simulink model "ITMBS_epushbtton_M0"  (R2023a)
settings: Solver=FixedStepDiscrete  StartTime=0.0  StopTime=10.0  FixedStep=0.05  RelTol=1e-3
libraries: legoev3lib x4
settings Model: Creator=kevin  LastModifiedBy=Sachin K S

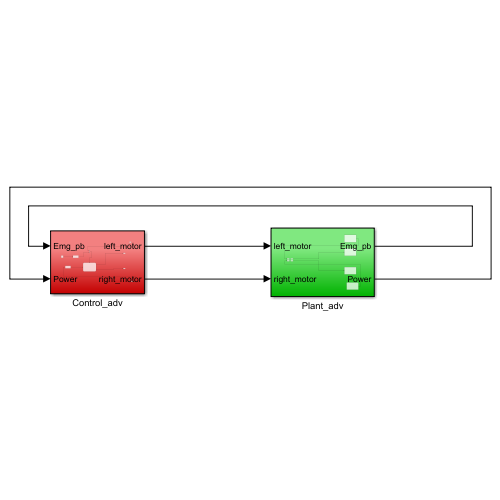
[thumbnail: Simulink's stored preview of the top-level diagram]
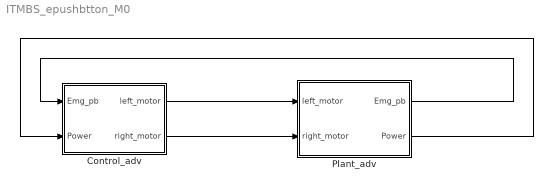
== system ITMBS_epushbtton_M0 ==
  Control_adv : Subsystem
  Plant_adv : Subsystem
  wires:
  Control_adv/1(left_motor) -> Plant_adv/1(left_motor)
  Control_adv/2(right_motor) -> Plant_adv/2(right_motor)
  Plant_adv/1(Emg_pb) -> Control_adv/1(Emg_pb)
  Plant_adv/2(Power) -> Control_adv/2(Power)

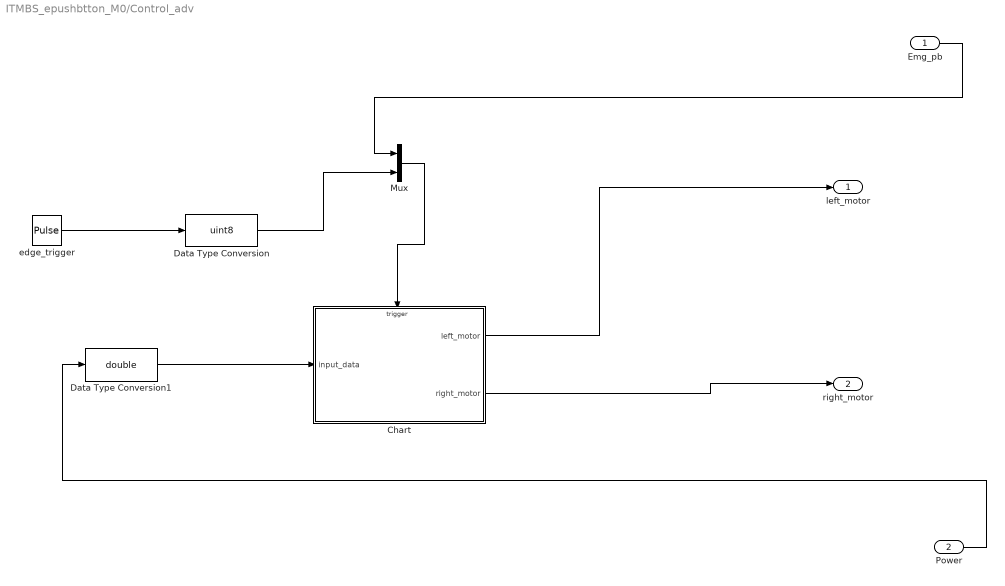
== system ITMBS_epushbtton_M0/Control_adv ==
  Emg_pb : Inport
  Power : Inport  Port=2
  Chart : Stateflow chart  TreatAsAtomicUnit=on
  Data Type Conversion : DataTypeConversion  OutDataTypeStr=uint8  SaturateOnIntegerOverflow=off  RndMeth=Floor
  Data Type Conversion1 : DataTypeConversion  OutDataTypeStr=double  SaturateOnIntegerOverflow=off  RndMeth=Floor
  Mux : Mux  Inputs=2
  edge_trigger : DiscretePulseGenerator  Period=3  PulseWidth=2  SampleTime=0.05
  left_motor : Outport
  right_motor : Outport  Port=2
  wires:
  Mux/1 -> Chart/Trigger
  edge_trigger/1 -> Data Type Conversion/1
  Chart/1(left_motor) -> left_motor/1
  Chart/2(right_motor) -> right_motor/1
  Data Type Conversion/1 -> Mux/2
  Data Type Conversion1/1 -> Chart/1(input_data)
  Power/1 -> Data Type Conversion1/1
  Emg_pb/1 -> Mux/1

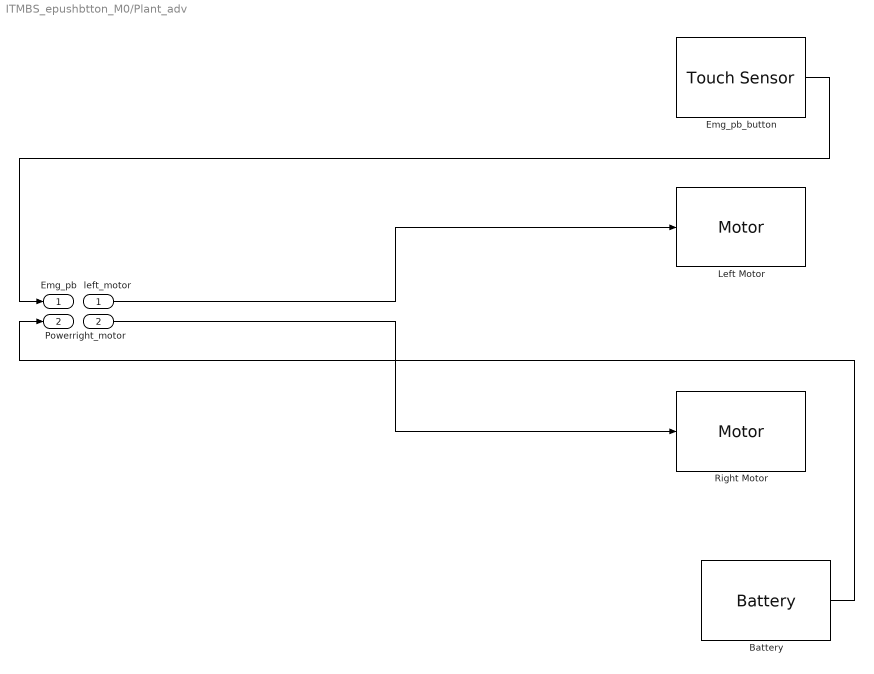
== system ITMBS_epushbtton_M0/Plant_adv ==
  left_motor : Inport
  right_motor : Inport  Port=2
  Battery : legoev3lib/Battery  SampleTime=0.1
  Emg_pb_button : legoev3lib/Touch Sensor  portNumber=1  sampleTime=0.1
  Left Motor : legoev3lib/Motor  sportNumber=A  sstopAction=Brake
  Right Motor : legoev3lib/Motor  sportNumber=A  sstopAction=Brake
  Emg_pb : Outport
  Power : Outport  Port=2
  wires:
  Emg_pb_button/1 -> Emg_pb/1
  left_motor/1 -> Left Motor/1
  right_motor/1 -> Right Motor/1
  Battery/1 -> Power/1

== stateflow chart ITMBS_epushbtton_M0/Control_adv/Chart ==
  settings: executeAtInitialization=1
  state On_Em
    right_motor = input_data;
    left_motor = input_data;
  state Off_Em
    right_motor=0;
    left_motor=0;
    entry:
    c=0;
  (default) -> On_Em
  On_Em -> Off_Em : [pushbutton_event_input ]
  (junction 38) -> On_Em [order 1] : [c==2]
  Off_Em -> (junction 36)
  (junction 36) -> (junction 37) [order 1] : [pushbutton_event_input]
  (junction 36) -> (junction 38) [order 2]
  (junction 37) -> (junction 39) : {c= c+1;}
  (junction 39) -> (junction 38)
  (junction 38) -> (junction 53) [order 2]
  data: input_data input; c local; left_motor output; right_motor output
  events: pushbutton_event_input input RISING_EDGE_EVENT; trigger input RISING_EDGE_EVENT
